simulink model "lab2_1"  (R2015b)
settings: Solver=VariableStepAuto  StartTime=0  StopTime=0.0015  RelTol=1e-3
values from neighbouring files (symbols this model uses):
  A = 1    [dev_digicomm_lab2.m]
  T = 1.5E-3    (= 0.0015)    [dev_digicomm_lab2.m]
  t0 = 0    [dev_digicomm_lab2.m]
  t1 = N1*T    (= 0.00015)    [dev_digicomm_lab2.m]
  t2 = (N1+N2)*T    (= 0.00045)    [dev_digicomm_lab2.m]
  t3 = (N1+N2+N3)*T    (= 0.000825)    [dev_digicomm_lab2.m]
  Ts = 1E-6    (= 1e-06)    [dev_digicomm_lab2.m]
libraries: simulink x1
settings Model: Creator=trejo  LastModifiedBy=trejo

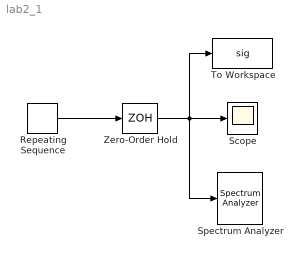
== system lab2_1 ==
  Repeating Sequence : simulink/Sources/Repeating Sequence  rep_seq_t=[t0 t1 t2 t3 T]  rep_seq_y=[0 A A 0 0]
  Scope : Scope
  Spectrum Analyzer : SpectrumAnalyzer
  To Workspace : ToWorkspace  VariableName=sig  SaveFormat=Timeseries  SampleTime=-1
  Zero-Order Hold : ZeroOrderHold  SampleTime=Ts
  wires:
  Repeating Sequence/1 -> Zero-Order Hold/1
  Zero-Order Hold/1 -> To Workspace/1, Spectrum Analyzer/1, Scope/1
